simulink model "DC_motor_drive_sim"  (R2019b)
settings: Solver=ode23t  StartTime=0.0  StopTime=end_time  RelTol=1e-3
values from neighbouring files (symbols this model uses):
  Ia_rated = 25    [DC_motor_init.m]
  J = 0.00252    [DC_motor_init.m]
  Power = 3336    [DC_motor_init.m]
  Wm_rated = 3000*(2*pi/60)    (= 314.159265359)    [DC_motor_init.m]
libraries: fl_lib x5, ee_lib x2, nesl_utility x2
settings Model: Creator=faaizz  LastModifiedBy=faaizz
settings SimscapeCC: SimscapeLogType=all  SimscapeLogSimulationStatistics=on

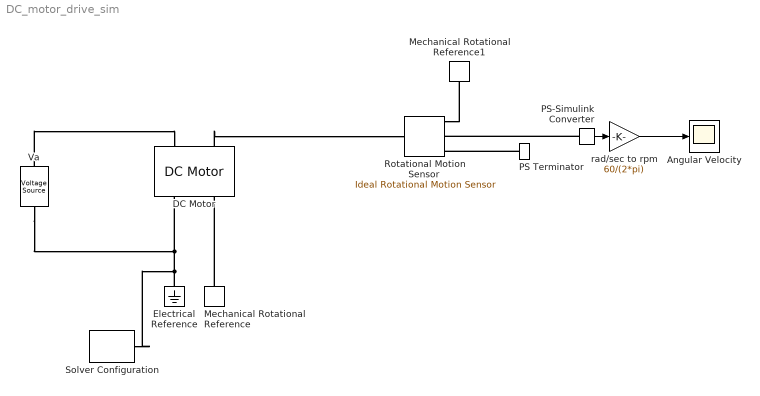
== system DC_motor_drive_sim ==
  Angular Velocity : Scope
  DC Motor : ee_lib/Electromechanical/Brushed Motors/DC Motor  parameterization=1  Ra=Ra Ohm  La=La H  emf_or_torque=2  Kv=0.072e-3 V/rpm  Ki=(Power/Wm_rated)/Ia_rated N*m/A  T_stall=0.24e-3 N*m  w_max=19100 rpm  w_rated=15000 rpm  P_rated=0.08 W  V_rated=1.5 V  J=J kg*m^2  lam_param=1  lam=B N*m/(rad/s)  i_noload=0 A  V_i_noload=1.5 V  speed0=0 rpm  alpha=3.93e-3 1/K  Tmeas=25 degC  thermal_mass=100 J/K  initial_temperature=25 degC
      settings: SourceProductName=Simscape Electrical
  Electrical Reference : fl_lib/Electrical/Electrical Elements/Electrical Reference
  Mechanical Rotational Reference : fl_lib/Mechanical/Rotational Elements/Mechanical Rotational Reference
  Mechanical Rotational Reference1 : fl_lib/Mechanical/Rotational Elements/Mechanical Rotational Reference
  PS Terminator : fl_lib/Physical Signals/Sinks/PS Terminator
      settings: SourceProductName=Simscape
  PS-Simulink Converter : nesl_utility/PS-Simulink Converter  PhysicalDomain=network_engine_domain  SubClassName=ps_output  LeftPortType=input  RightPortType=output  PseudoPeriodic=off  Frequencies=[]  Unit=inherit  AffineConversion=off
  Rotational Motion Sensor : fl_lib/Mechanical/Mechanical Sensors/Ideal Rotational Motion Sensor  offset=0 rev
  Solver Configuration : nesl_utility/Solver Configuration  PhysicalDomain=network_engine_domain  SubClassName=solver  LeftPortType=input  RightPortType=generic  Tones=[]  Harmonics=[]  SimulateNoise=off  Profile=off  UseLocalSampling=off  EnableSwitchedLinearOptims=on  FrequencyDomain=off  UseCCode=off  RelTol=0.001  AbsTol=1e-06  MinStep=1e-09  ToWorkspace=off  RevertToSquareIcSolve=off  NumHomotopyIterations=100  PhasorMode=off  PhasorModeNumHarmonics=1  DoDC=off  ResidualTolerance=1e-09  UseLocalSolver=off  LocalSolverChoice=NE_BACKWARD_EULER_ADVANCER  LocalSolverSampleTime=0.001  DoFixedCost=off  MaxNonlinIter=3  MaxModeIter=2  LinearAlgebra=auto  EquationFormulation=NE_TIME_EF  DelaysMemoryBudget=1024  AutomaticFiltering=on  FilteringTimeConstant=0.001  PartitionStorageMethod=AS_NEEDED  PartitionMemoryBudget=1024  PartitionMethod=ROBUST
  Va : ee_lib/Sources/Voltage Source  dc_voltage=Va V  ac_voltage=0 V  ac_shift=0 rad  ac_frequency=60 Hz  noise_mode=0  PSD=0 V^2/Hz  repeatability=1  auto_seed=725806650  user_seed=0  sample_time=1e-3 s  i_specify=off  i_priority=None  i=0 A  i_nominal_specify=off  i_nominal_unit=A  i_nominal_value=1  v_specify=off  v_priority=None  v=0 V  v_nominal_specify=off  v_nominal_unit=V  v_nominal_value=1
      settings: SourceProductName=Simscape Electrical
  rad/sec to rpm : Gain  Gain=60/(2*pi)
  wires:
  PS-Simulink Converter/1 -> rad/sec to rpm/1
  rad/sec to rpm/1 -> Angular Velocity/1
  connections:
  Mechanical Rotational Reference/LConn1 -- DC Motor/RConn2
  Electrical Reference/LConn1 -- Solver Configuration/RConn1 -- Va/RConn1 -- DC Motor/RConn1
  DC Motor/LConn2 -- Rotational Motion Sensor/LConn1
  Rotational Motion Sensor/RConn1 -- Mechanical Rotational Reference1/LConn1
  PS-Simulink Converter/LConn1 -- Rotational Motion Sensor/RConn2
  PS Terminator/LConn1 -- Rotational Motion Sensor/RConn3
  Va/LConn1 -- DC Motor/LConn1
